simulink model "validate_gyro"  (R2014a)
settings: Solver=VariableStepDiscrete  StartTime=0.0  StopTime=t_sim  MaxStep=0.001  RelTol=1e-3
undefined symbols (not defined in the file): diff, gyro_data, omega_bias_I_noise, R_gyro
libraries: lib_gyro_fusion x7
settings Model: Creator=kirill  LastModifiedBy=kirill

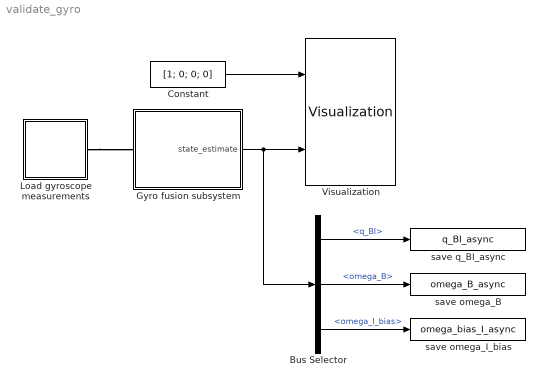
== system validate_gyro ==
  Bus Selector : BusSelector  OutputSignals=q_BI,omega_B,omega_I_bias
  Constant : Constant  Value=[1; 0; 0; 0]
  Gyro fusion subsystem : Subsystem
  Load gyroscope measurements : Subsystem  mask{measurement_type=1, observed_data=gyro_data, R_measurement=R_gyro}
      mask prompts: measurement_type "Measuerment type (integer identifyer)"; observed_data "Observation data (see from workspace documentation)"; R_measurement "Measurement covariance matrix"
  Visualization : lib_gyro_fusion/Visualization
  save omega_B : ToWorkspace  VariableName=omega_B_async  SaveFormat=Timeseries  SampleTime=-1
  save omega_I_bias : ToWorkspace  VariableName=omega_bias_I_async  SaveFormat=Timeseries  SampleTime=-1
  save q_BI_async : ToWorkspace  VariableName=q_BI_async  SaveFormat=Timeseries  SampleTime=-1
  wires:
  Gyro fusion subsystem/1(state_estimate) -> Visualization/2, Bus Selector/1
  Constant/1 -> Visualization/1
  Bus Selector/1 -> save q_BI_async/1  "<q_BI>"
  Bus Selector/3 -> save omega_I_bias/1  "<omega_I_bias>"
  Bus Selector/2 -> save omega_B/1  "<omega_B>"
  connections:
  Load gyroscope measurements/RConn1 -- Gyro fusion subsystem/LConn1

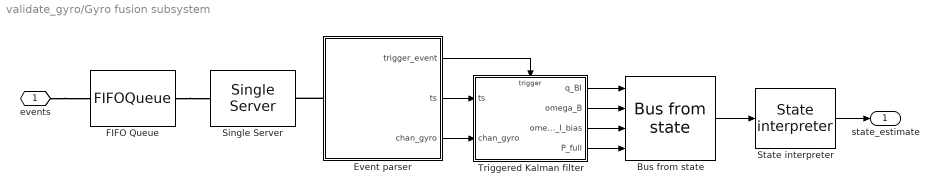
== system validate_gyro/Gyro fusion subsystem ==
  Bus from state : lib_gyro_fusion/Bus from state
  Event parser : Subsystem
  FIFO Queue : FIFOQueue  Capacity=500
  Single Server : SingleServer  ServiceTime=0.001
  State interpreter : lib_gyro_fusion/State interpreter
  Triggered Kalman filter : Subsystem  TreatAsAtomicUnit=on
  events : PMIOPort  Port=1  Side=Left
  state_estimate : Outport
  wires:
  Event parser/3(chan_gyro) -> Triggered Kalman filter/2(chan_gyro)
  State interpreter/1 -> state_estimate/1
  Event parser/1(trigger_event) -> Triggered Kalman filter/Trigger
  Event parser/2(ts) -> Triggered Kalman filter/1(ts)
  Triggered Kalman filter/1(q_BI) -> Bus from state/1
  Triggered Kalman filter/2(omega_B) -> Bus from state/2
  Triggered Kalman filter/3(omega_I_bias) -> Bus from state/3
  Triggered Kalman filter/4(P_full) -> Bus from state/4
  Bus from state/1 -> State interpreter/1
  connections:
  events/RConn1 -- FIFO Queue/LConn1
  FIFO Queue/RConn1 -- Single Server/LConn1
  Event parser/LConn1 -- Single Server/RConn1

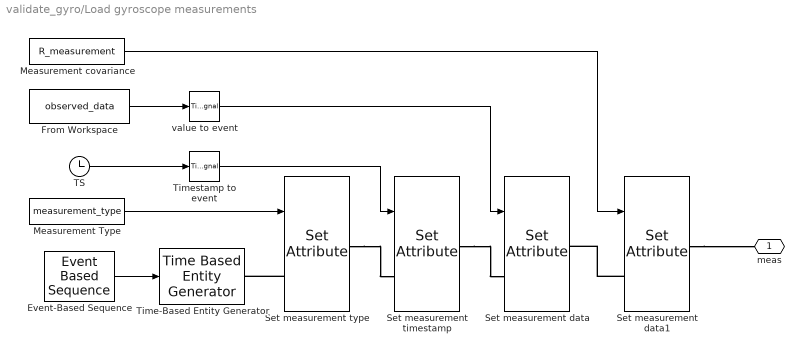
== system validate_gyro/Load gyroscope measurements ==
  Event-Based Sequence : EventBasedSequence  VectorOutputValues=diff(observed_data.time)  FormOutputOpt=Setting to infinity
  From Workspace : FromWorkspace  VariableName=observed_data  SampleTime=0
  Measurement Type : Constant  Value=measurement_type
  Measurement covariance : Constant  Value=R_measurement
  Set measurement data : SetAttribute  AttributeName=value  AttributeFrom=Signal port  EvaluatedAttributeValue={ []}
  Set measurement data1 : SetAttribute  AttributeName=R  AttributeFrom=Signal port  EvaluatedAttributeValue={ []}
  Set measurement timestamp : SetAttribute  AttributeName=ts  AttributeFrom=Signal port  EvaluatedAttributeValue={ []}
  Set measurement type : SetAttribute  AttributeName=meas_type  AttributeFrom=Signal port  EvaluatedAttributeValue={ []}
  TS : Clock
  Time-Based Entity Generator : TimeBasedEntityGenerator  GenerateEntitiesUpon=Intergeneration time from port t
  Timestamp to event : TimedToEventSignal
  value to event : TimedToEventSignal
  meas : PMIOPort  Port=1  Side=Right
  wires:
  TS/1 -> Timestamp to event/1
  From Workspace/1 -> value to event/1
  Event-Based Sequence/1 -> Time-Based Entity Generator/1
  Measurement Type/1 -> Set measurement type/1
  Timestamp to event/1 -> Set measurement timestamp/1
  value to event/1 -> Set measurement data/1
  Measurement covariance/1 -> Set measurement data1/1
  connections:
  Set measurement type/LConn1 -- Time-Based Entity Generator/RConn1
  Set measurement data1/RConn1 -- meas/RConn1
  Set measurement type/RConn1 -- Set measurement timestamp/LConn1
  Set measurement timestamp/RConn1 -- Set measurement data/LConn1
  Set measurement data1/LConn1 -- Set measurement data/RConn1

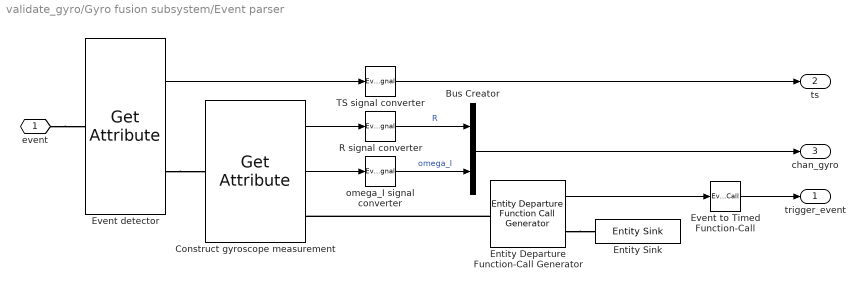
== system validate_gyro/Gyro fusion subsystem/Event parser ==
  Bus Creator : BusCreator  Inputs=2
  Construct gyroscope measurement : GetAttribute  AttributeName=R|value  AttributeMissing=Error|Error  AttributeDefaultValue=1|1  AttributeTreatAsVector=1|1  AttributeSendTiming=After entity departure|After entity departure  EvaluatedDefaultAttributeValue={ [];[]}
      settings: OutputPortMap=o1,o2
  Entity Departure Function-Call Generator : EntityDepartureFunctionCallGenerator
  Entity Sink : EntitySink
  Event detector : GetAttribute  AttributeName=ts  EvaluatedDefaultAttributeValue={ []}
      settings: OutputPortMap=o1
  Event to Timed Function-Call : EventToTimedFunctionCall
  R signal converter : EventToTimedSignal
  TS signal converter : EventToTimedSignal
  omega_I signal converter : EventToTimedSignal
  event : PMIOPort  Port=1  Side=Left
  trigger_event : Outport
  ts : Outport  Port=2
  chan_gyro : Outport  Port=3
  wires:
  Construct gyroscope measurement/2 -> omega_I signal converter/1
  Construct gyroscope measurement/1 -> R signal converter/1
  Bus Creator/1 -> chan_gyro/1
  R signal converter/1 -> Bus Creator/1  "R"
  omega_I signal converter/1 -> Bus Creator/2  "omega_I"
  Entity Departure Function-Call Generator/1 -> Event to Timed Function-Call/1
  Event to Timed Function-Call/1 -> trigger_event/1
  TS signal converter/1 -> ts/1
  Event detector/1 -> TS signal converter/1
  connections:
  Entity Departure Function-Call Generator/LConn1 -- Construct gyroscope measurement/RConn1
  Event detector/RConn1 -- Construct gyroscope measurement/LConn1
  Entity Departure Function-Call Generator/RConn1 -- Entity Sink/LConn1
  event/RConn1 -- Event detector/LConn1

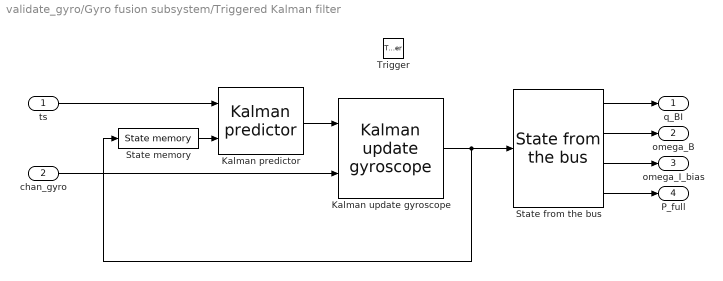
== system validate_gyro/Gyro fusion subsystem/Triggered Kalman filter ==
  ts : Inport
  chan_gyro : Inport  Port=2
  Trigger : TriggerPort  TriggerType=function-call
  Kalman predictor : lib_gyro_fusion/Kalman predictor  q_noise=q_noise  omega_B_noise=omega_B_noise  omega_I_bias_noise=omega_bias_I_noise * 0
  Kalman update gyroscope : lib_gyro_fusion/Kalman update gyroscope
  State from the bus : lib_gyro_fusion/State from the bus
  State memory : lib_gyro_fusion/State memory  q_BI_init=[1; 0; 0; 0]  omega_B_init=[0; 0; 0]  omega_I_bias_init=[0; 0; 0]  P_full_init=eye(9) / 1e6
  q_BI : Outport
  omega_B : Outport  Port=2
  omega_I_bias : Outport  Port=3
  P_full : Outport  Port=4
  wires:
  ts/1 -> Kalman predictor/1
  chan_gyro/1 -> Kalman update gyroscope/2
  State memory/1 -> Kalman predictor/2
  Kalman update gyroscope/1 -> State memory/1, State from the bus/1
  Kalman predictor/1 -> Kalman update gyroscope/1
  State from the bus/1 -> q_BI/1
  State from the bus/4 -> P_full/1
  State from the bus/3 -> omega_I_bias/1
  State from the bus/2 -> omega_B/1
